simulink model "test_sim"  (Simulink 10.3)
settings: Solver=FixedStepAuto  StartTime=0.0  StopTime=3  FixedStep=0.0001  RelTol=1e-3  EnableMultiTasking=on
settings Model: Creator=ljk  LastModifiedBy=fu  ExtModeTrigMode=oneshot  ExtModeArmWhenConnect=off
settings OptimizationCC: BlockReduction=off  BooleanDataType=off
settings DebuggingCC: SaveWithParameterizedLinksMsg=none  SignalResolutionControl=TryResolveAllWithWarning  MultiTaskDSMMsg=warning  MultiTaskCondExecSysMsg=none
settings HardwareCC: TargetUnknown=on

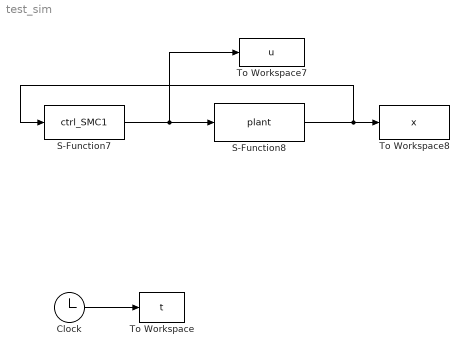
== system test_sim ==
  Clock : Clock
  S-Function7 : S-Function  FunctionName=ctrl_SMC1  SFunctionDeploymentMode=off  EnableBusSupport=off
  S-Function8 : S-Function  FunctionName=plant  SFunctionDeploymentMode=off  EnableBusSupport=off
  To Workspace : ToWorkspace  VariableName=t  SampleTime=-1
  To Workspace7 : ToWorkspace  VariableName=u  SampleTime=-1
  To Workspace8 : ToWorkspace  VariableName=x  SampleTime=-1
  wires:
  Clock/1 -> To Workspace/1
  S-Function8/1 -> S-Function7/1, To Workspace8/1
  S-Function7/1 -> S-Function8/1, To Workspace7/1
